simulink model "lqr_control"  (R2021a)
settings: Solver=FixedStepDiscrete  StartTime=0.0  StopTime=100  FixedStep=1e-02  RelTol=1e-3
values from neighbouring files (symbols this model uses):
  A = [0 1 ; 0 -Br/I]    [init.m]    (also in simple-init.m)
  B = [0 ;1]    [init.m]    (also in simple-init.m = [B(:,2)])
  C = [1 0]    [init.m]    (also in simple-init.m)
  g = 9.81    [init.m]    (also in simple-init.m)
  I = I1 + I2    (= 0.783146666667)    [init.m]    (also in simple-init.m = 0.698213333333)
  K = lqr(A,B,Q,R)    [init.m]    (also in simple-init.m)
  l1o = 0.07    [init.m]
  l2f = (l1 + l2)/2 + l3f + l3o    (= 0.65)    [init.m]    (also in simple-init.m = 0.62)
  l3f = l3o + 0.15    (= 0.3)    [init.m]    (also in simple-init.m)
  l3o = 0.15    [init.m]    (also in simple-init.m)
  m1 = 12    [init.m]    (also in simple-init.m = 3.92)
  m2 = 1.4    [init.m]    (also in simple-init.m = 1.7)
  x0 = [pi/8;0]    [init.m]    (also in simple-init.m)
undefined symbols (not defined in the file or in its folder): DiscIntNeverNeededParam
libraries: simulink x15
settings Model: Creator=DANI-TUF  LastModifiedBy=DANI-TUF

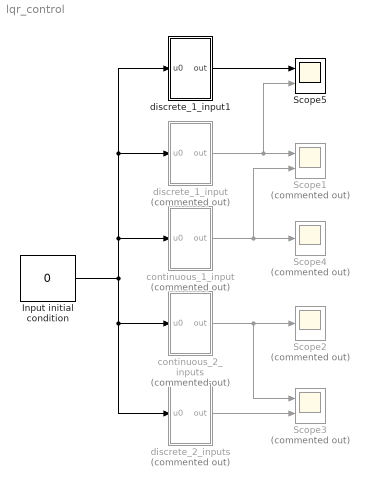
== system lqr_control ==
  Input initial condition : Constant  Value=0
  Scope1 : Scope  Commented=on  NumInputPorts=2
  Scope2 : Scope  Commented=on
  Scope3 : Scope  Commented=on  NumInputPorts=2
  Scope4 : Scope  Commented=on
  Scope5 : Scope  NumInputPorts=2
  continuous_1_input : Subsystem  Commented=on
  continuous_2_inputs : Subsystem  Commented=on
  discrete_1_input : Subsystem  Commented=on
  discrete_1_input1 : Subsystem
  discrete_2_inputs : Subsystem  Commented=on
  wires:
  continuous_2_inputs/1(out) -> Scope3/1, Scope2/1
  discrete_2_inputs/1(out) -> Scope3/2
  continuous_1_input/1(out) -> Scope1/2, Scope4/1
  discrete_1_input/1(out) -> Scope5/2, Scope1/1
  Input initial condition/1 -> continuous_2_inputs/1(u0), discrete_2_inputs/1(u0), discrete_1_input1/1(u0), discrete_1_input/1(u0), continuous_1_input/1(u0)
  discrete_1_input1/1(out) -> Scope5/1

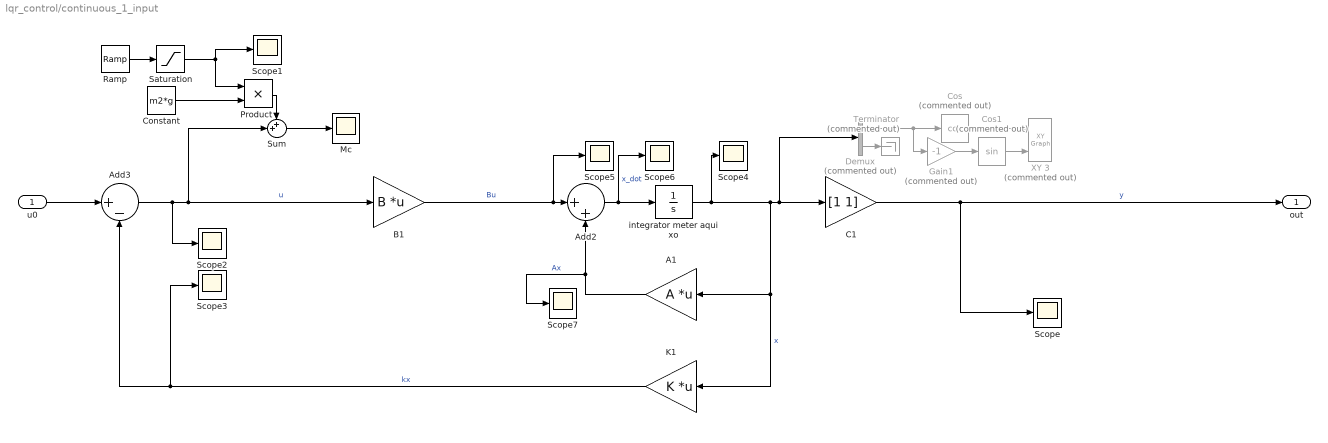
== system lqr_control/continuous_1_input ==
  u0 : Inport
  A1 : Gain  Gain=A  Multiplication=Matrix(K*u)
  Add2 : Sum  Inputs=|++
  Add3 : Sum  Inputs=|+-
  B1 : Gain  Gain=B  Multiplication=Matrix(K*u)
  C1 : Gain  Gain=[1 1]
  Constant : Constant  Value=m2*g
  Cos : Trigonometry  Commented=on  Operator=cos
  Cos1 : Trigonometry  Commented=on
  Demux : Demux  Commented=on  Outputs=2
  Gain1 : Gain  Commented=on  Gain=-1
  K1 : Gain  Gain=K  Multiplication=Matrix(K*u)
  Mc : Scope
  Product : Product
  Ramp : simulink/Sources/Ramp  slope=0.025  start=5  InitialOutput=l2f+l3o-l3f
  Saturation : Saturate  UpperLimit=l2f
  Scope{,1..7} (8 alike) : Scope
  Sum : Sum  Inputs=++|
  Terminator : Terminator  Commented=on
  XY 3 : simulink/Sinks/XY Graph  Commented=on  xmin=-2  xmax=2  ymin=-2  ymax=2  st=-1
  integrator meter aqui xo : Integrator  InitialCondition=x0
  out : Outport
  wires:
  Demux/2 -> Terminator/1
  C1/1 -> Scope/1, out/1  "y"
  Cos/1 -> XY 3/1
  Cos1/1 -> XY 3/2
  A1/1 -> Add2/2, Scope7/1  "Ax"
  u0/1 -> Add3/1
  B1/1 -> Add2/1, Scope5/1  "Bu"
  integrator meter aqui xo/1 -> A1/1, K1/1, Demux/1, C1/1, Scope4/1  "x"
  Add2/1 -> integrator meter aqui xo/1, Scope6/1  "x_dot"
  K1/1 -> Scope3/1, Add3/2  "kx"
  Add3/1 -> Scope2/1, Sum/2, B1/1  "u"
  Gain1/1 -> Cos1/1
  Demux/1 -> Gain1/1, Cos/1
  Sum/1 -> Mc/1
  Constant/1 -> Product/2
  Ramp/1 -> Saturation/1
  Saturation/1 -> Product/1, Scope1/1
  Product/1 -> Sum/1

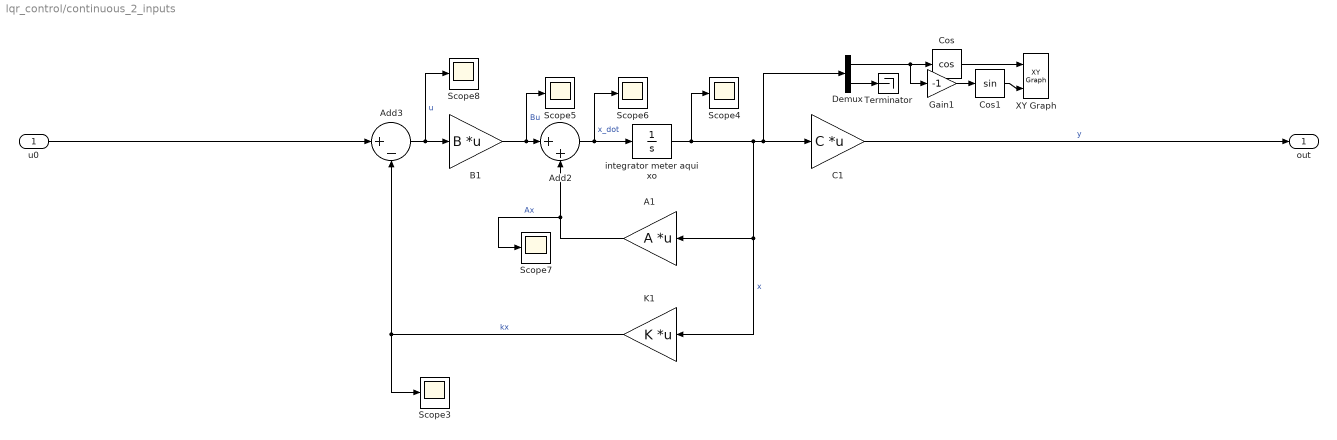
== system lqr_control/continuous_2_inputs ==
  u0 : Inport
  A1 : Gain  Gain=A  Multiplication=Matrix(K*u)
  Add2 : Sum  Inputs=|++
  Add3 : Sum  Inputs=|+-
  B1 : Gain  Gain=B  Multiplication=Matrix(K*u)
  C1 : Gain  Gain=C  Multiplication=Matrix(K*u)
  Cos : Trigonometry  Operator=cos
  Cos1 : Trigonometry
  Demux : Demux  Outputs=2
  Gain1 : Gain  Gain=-1
  K1 : Gain  Gain=K  Multiplication=Matrix(K*u)
  Scope{3..8} (6 alike) : Scope
  Terminator : Terminator
  XY Graph : simulink/Sinks/XY Graph  xmin=-2  xmax=2  ymin=-2  ymax=2  st=-1
  integrator meter aqui xo : Integrator  InitialCondition=[pi/16; 0]
  out : Outport
  wires:
  K1/1 -> Add3/2, Scope3/1  "kx"
  Add2/1 -> Scope6/1, integrator meter aqui xo/1  "x_dot"
  Demux/1 -> Gain1/1, Cos/1
  integrator meter aqui xo/1 -> Scope4/1, Demux/1, C1/1, K1/1, A1/1  "x"
  B1/1 -> Scope5/1, Add2/1  "Bu"
  Add3/1 -> Scope8/1, B1/1  "u"
  u0/1 -> Add3/1
  A1/1 -> Scope7/1, Add2/2  "Ax"
  Cos1/1 -> XY Graph/2
  Cos/1 -> XY Graph/1
  C1/1 -> out/1  "y"
  Demux/2 -> Terminator/1
  Gain1/1 -> Cos1/1

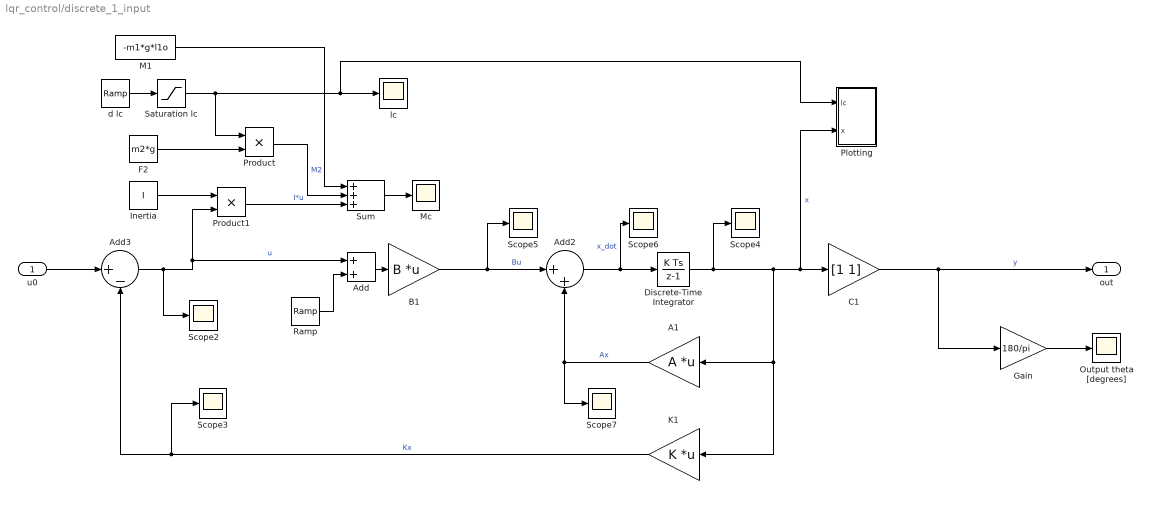
== system lqr_control/discrete_1_input ==
  u0 : Inport
  A1 : Gain  Gain=A  Multiplication=Matrix(K*u)
  Add : Sum
  Add2 : Sum  Inputs=|++
  Add3 : Sum  Inputs=|+-
  B1 : Gain  Gain=B  Multiplication=Matrix(K*u)
  C1 : Gain  Gain=[1 1]
  Discrete-Time Integrator : DiscreteIntegrator  InitialCondition=x0  SampleTime=1e-3  ICPrevOutput=DiscIntNeverNeededParam  ICPrevScaledInput=DiscIntNeverNeededParam
  F2 : Constant  Value=m2*g
  Gain : Gain  Gain=180/pi
  Inertia : Constant  Value=I
  K1 : Gain  Gain=K  Multiplication=Matrix(K*u)
  M1 : Constant  Value=-m1*g*l1o
  Mc : Scope
  Output theta [degrees] : Scope
  Plotting : Subsystem
  Product : Product
  Product1 : Product
  Ramp : simulink/Sources/Ramp  slope=1  start=25  InitialOutput=0
  Saturation lc : Saturate  UpperLimit=l2f
  Scope{2..7} (6 alike) : Scope
  Sum : Sum  Inputs=+++
  d lc : simulink/Sources/Ramp  slope=0.025  start=15  InitialOutput=l2f+l3o-l3f
  lc : Scope
  out : Outport
  wires:
  Saturation lc/1 -> Plotting/1(lc), lc/1, Product/1
  d lc/1 -> Saturation lc/1
  F2/1 -> Product/2
  Sum/1 -> Mc/1
  Add3/1 -> Add/1, Product1/2, Scope2/1  "u"
  K1/1 -> Add3/2, Scope3/1  "Kx"
  Add2/1 -> Discrete-Time Integrator/1, Scope6/1  "x_dot"
  Discrete-Time Integrator/1 -> Scope4/1, Plotting/2(x), C1/1, K1/1, A1/1  "x"
  B1/1 -> Add2/1, Scope5/1  "Bu"
  u0/1 -> Add3/1
  A1/1 -> Add2/2, Scope7/1  "Ax"
  C1/1 -> out/1, Gain/1  "y"
  Gain/1 -> Output theta [degrees]/1
  Inertia/1 -> Product1/1
  Product1/1 -> Sum/3  "I*u"
  M1/1 -> Sum/1
  Product/1 -> Sum/2  "M2"
  Ramp/1 -> Add/2
  Add/1 -> B1/1

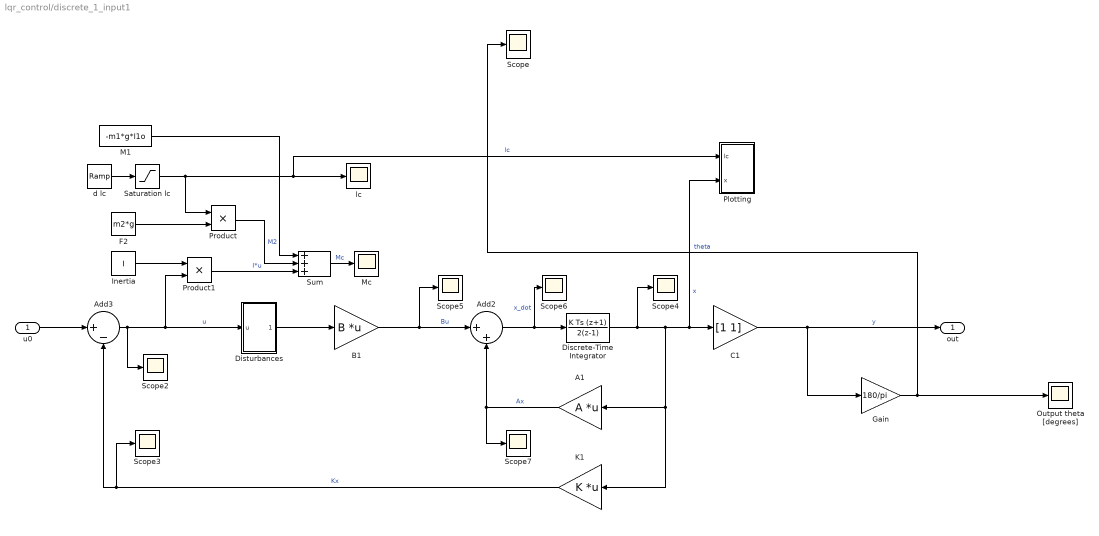
== system lqr_control/discrete_1_input1 ==
  u0 : Inport
  A1 : Gain  Gain=A  Multiplication=Matrix(K*u)
  Add2 : Sum  Inputs=|++
  Add3 : Sum  Inputs=|+-
  B1 : Gain  Gain=B  Multiplication=Matrix(K*u)
  C1 : Gain  Gain=[1 1]
  Discrete-Time Integrator : DiscreteIntegrator  IntegratorMethod=Integration: Trapezoidal  InitialCondition=x0  SampleTime=-1  ICPrevOutput=DiscIntNeverNeededParam  ICPrevScaledInput=DiscIntNeverNeededParam
  Disturbances : Subsystem
  F2 : Constant  Value=m2*g
  Gain : Gain  Gain=180/pi
  Inertia : Constant  Value=I
  K1 : Gain  Gain=K  Multiplication=Matrix(K*u)
  M1 : Constant  Value=-m1*g*l1o
  Mc : Scope
  Output theta [degrees] : Scope
  Plotting : Subsystem
  Product : Product
  Product1 : Product
  Saturation lc : Saturate  UpperLimit=l2f
  Scope{,2..7} (7 alike) : Scope
  Sum : Sum  Inputs=+++
  d lc : simulink/Sources/Ramp  slope=0.025  start=12  InitialOutput=l2f+l3o-l3f
  lc : Scope
  out : Outport
  wires:
  Product/1 -> Sum/2  "M2"
  M1/1 -> Sum/1
  Product1/1 -> Sum/3  "I*u"
  Inertia/1 -> Product1/1
  Gain/1 -> Scope/1, Output theta [degrees]/1  "theta"
  C1/1 -> Gain/1, out/1  "y"
  A1/1 -> Scope7/1, Add2/2  "Ax"
  u0/1 -> Add3/1
  B1/1 -> Scope5/1, Add2/1  "Bu"
  Discrete-Time Integrator/1 -> A1/1, K1/1, C1/1, Plotting/2(x), Scope4/1  "x"
  Add2/1 -> Discrete-Time Integrator/1, Scope6/1  "x_dot"
  K1/1 -> Scope3/1, Add3/2  "Kx"
  Add3/1 -> Product1/2, Disturbances/1(u), Scope2/1  "u"
  Sum/1 -> Mc/1  "Mc"
  F2/1 -> Product/2
  d lc/1 -> Saturation lc/1
  Saturation lc/1 -> Product/1, lc/1, Plotting/1(lc)  "lc"
  Disturbances/1(u + dist) -> B1/1

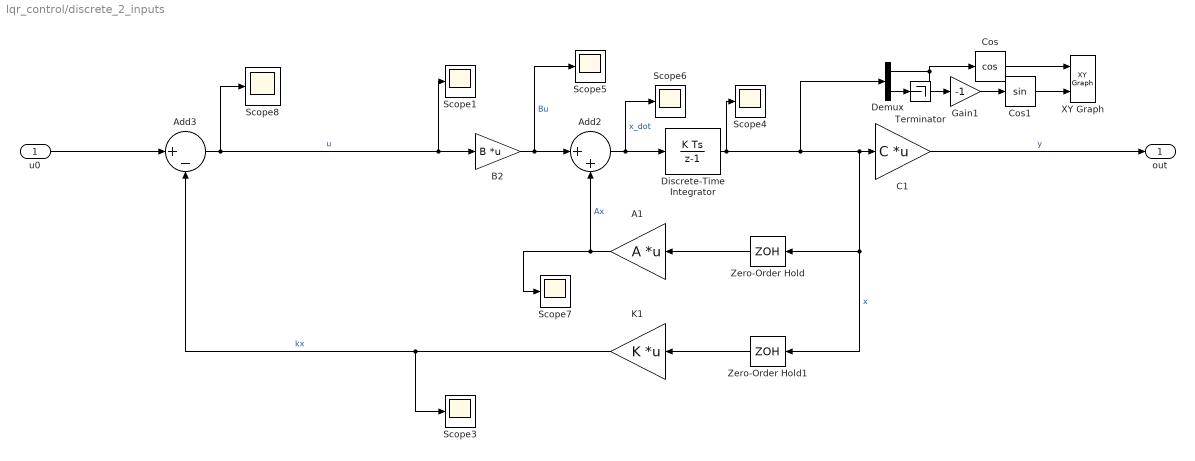
== system lqr_control/discrete_2_inputs ==
  u0 : Inport
  A1 : Gain  Gain=A  Multiplication=Matrix(K*u)
  Add2 : Sum  Inputs=|++
  Add3 : Sum  Inputs=|+-
  B2 : Gain  Gain=B  Multiplication=Matrix(K*u)
  C1 : Gain  Gain=C  Multiplication=Matrix(K*u)
  Cos : Trigonometry  Operator=cos
  Cos1 : Trigonometry
  Demux : Demux  Outputs=2
  Discrete-Time Integrator : DiscreteIntegrator  InitialCondition=[pi/16 ;0]  SampleTime=1e-3  ICPrevOutput=DiscIntNeverNeededParam  ICPrevScaledInput=DiscIntNeverNeededParam
  Gain1 : Gain  Gain=-1
  K1 : Gain  Gain=K  Multiplication=Matrix(K*u)
  Scope{1,3..8} (7 alike) : Scope
  Terminator : Terminator
  XY Graph : simulink/Sinks/XY Graph  xmin=-2  xmax=2  ymin=-2  ymax=2  st=-1
  Zero-Order Hold : ZeroOrderHold  SampleTime=1e-3
  Zero-Order Hold1 : ZeroOrderHold  SampleTime=1e-3
  out : Outport
  wires:
  Demux/2 -> Terminator/1
  C1/1 -> out/1  "y"
  Cos/1 -> XY Graph/1
  Cos1/1 -> XY Graph/2
  A1/1 -> Add2/2, Scope7/1  "Ax"
  u0/1 -> Add3/1
  Add3/1 -> Scope1/1, B2/1, Scope8/1  "u"
  Discrete-Time Integrator/1 -> Demux/1, Zero-Order Hold/1, Zero-Order Hold1/1, C1/1, Scope4/1  "x"
  Demux/1 -> Cos/1, Gain1/1
  Add2/1 -> Discrete-Time Integrator/1, Scope6/1  "x_dot"
  K1/1 -> Scope3/1, Add3/2  "kx"
  Zero-Order Hold/1 -> A1/1
  Zero-Order Hold1/1 -> K1/1
  B2/1 -> Scope5/1, Add2/1  "Bu"
  Gain1/1 -> Cos1/1

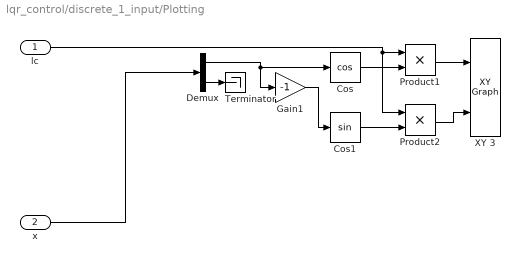
== system lqr_control/discrete_1_input/Plotting ==
  lc : Inport
  x : Inport  Port=2
  Cos : Trigonometry  Operator=cos
  Cos1 : Trigonometry
  Demux : Demux  Outputs=2
  Gain1 : Gain  Gain=-1
  Product1 : Product
  Product2 : Product
  Terminator : Terminator
  XY 3 : simulink/Sinks/XY Graph  xmin=-1  xmax=1  ymin=-1  ymax=1  st=-1
  wires:
  Demux/2 -> Terminator/1
  Cos/1 -> Product1/2
  Demux/1 -> Cos/1, Gain1/1
  Product2/1 -> XY 3/2
  Cos1/1 -> Product2/2
  lc/1 -> Product2/1, Product1/1
  Gain1/1 -> Cos1/1
  Product1/1 -> XY 3/1
  x/1 -> Demux/1

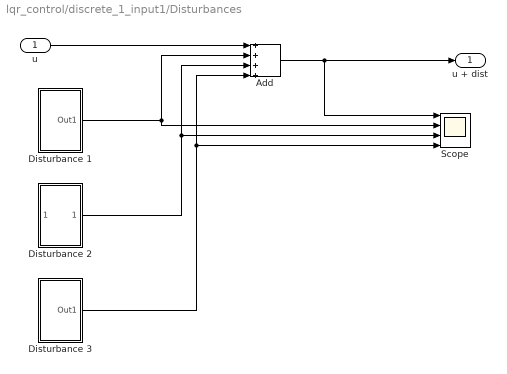
== system lqr_control/discrete_1_input1/Disturbances ==
  u : Inport
  Add : Sum  Inputs=++++
  Disturbance 1 : Subsystem
  Disturbance 2 : Subsystem
  Disturbance 3 : Subsystem
  Scope : Scope  NumInputPorts=4
  u + dist : Outport
  wires:
  Add/1 -> u + dist/1, Scope/1
  Disturbance 1/1(Out1) -> Scope/2, Add/2
  Disturbance 2/1(Out1) -> Add/3, Scope/3
  u/1 -> Add/1
  Disturbance 3/1(Out1) -> Scope/4, Add/4

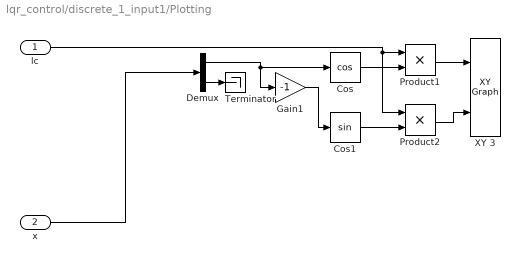
== system lqr_control/discrete_1_input1/Plotting ==
  lc : Inport
  x : Inport  Port=2
  Cos : Trigonometry  Operator=cos
  Cos1 : Trigonometry
  Demux : Demux  Outputs=2
  Gain1 : Gain  Gain=-1
  Product1 : Product
  Product2 : Product
  Terminator : Terminator
  XY 3 : simulink/Sinks/XY Graph  xmin=-1  xmax=1  ymin=-1  ymax=1  st=-1
  wires:
  x/1 -> Demux/1
  Product1/1 -> XY 3/1
  Gain1/1 -> Cos1/1
  lc/1 -> Product1/1, Product2/1
  Cos1/1 -> Product2/2
  Product2/1 -> XY 3/2
  Demux/1 -> Gain1/1, Cos/1
  Cos/1 -> Product1/2
  Demux/2 -> Terminator/1

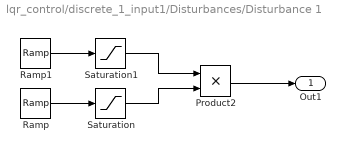
== system lqr_control/discrete_1_input1/Disturbances/Disturbance 1 ==
  Product2 : Product
  Ramp : simulink/Sources/Ramp  slope=0.003  start=18  InitialOutput=0
  Ramp1 : simulink/Sources/Ramp  slope=-1  start=28  InitialOutput=1
  Saturation : Saturate  UpperLimit=1  LowerLimit=-inf
  Saturation1 : Saturate  UpperLimit=1  LowerLimit=0
  Out1 : Outport
  wires:
  Saturation/1 -> Product2/2
  Ramp1/1 -> Saturation1/1
  Product2/1 -> Out1/1
  Ramp/1 -> Saturation/1
  Saturation1/1 -> Product2/1

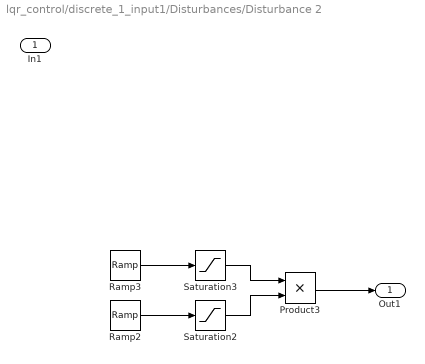
== system lqr_control/discrete_1_input1/Disturbances/Disturbance 2 ==
  In1 : Inport
  Product3 : Product
  Ramp2 : simulink/Sources/Ramp  slope=0.02  start=50  InitialOutput=0
  Ramp3 : simulink/Sources/Ramp  slope=-1  start=60  InitialOutput=1
  Saturation2 : Saturate  UpperLimit=1  LowerLimit=-inf
  Saturation3 : Saturate  UpperLimit=2  LowerLimit=0
  Out1 : Outport
  wires:
  Saturation3/1 -> Product3/1
  Ramp2/1 -> Saturation2/1
  Saturation2/1 -> Product3/2
  Ramp3/1 -> Saturation3/1
  Product3/1 -> Out1/1

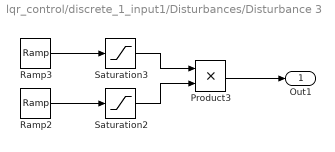
== system lqr_control/discrete_1_input1/Disturbances/Disturbance 3 ==
  Product3 : Product
  Ramp2 : simulink/Sources/Ramp  slope=-0.02  start=74  InitialOutput=0
  Ramp3 : simulink/Sources/Ramp  slope=-1  start=80  InitialOutput=1
  Saturation2 : Saturate  UpperLimit=inf  LowerLimit=-5
  Saturation3 : Saturate  UpperLimit=inf  LowerLimit=0
  Out1 : Outport
  wires:
  Product3/1 -> Out1/1
  Ramp3/1 -> Saturation3/1
  Saturation2/1 -> Product3/2
  Ramp2/1 -> Saturation2/1
  Saturation3/1 -> Product3/1
